simulink model "ACAES"  (R2026a)
settings: Solver=ode45  StopTime=t_sim_end  MaxStep=dt  MinStep=1  AbsTol=1e-6
model workspace (MAT data in the model file):
  Constant_mdot_ctrl = 0
  P0 = 101325
  P_comp_rated_W = 100000
  P_turb_rated_W = 100000
  T0 = 293.15
  buy_price = 15
  m_dot_chg_nom = 0.5
  m_dot_dis_nom = 0.6
  sell_price = 10
values from neighbouring files (symbols this model uses):
  cp_air = 1005.0    (= 1005)    [ACAES_params.m]    (also in ACAES_params.mat; CAES_init.m; IDKWHATTHISIS.mat)
  cp_TES = 2000    [ACAES_params.m]    (also in ACAES_params.mat; CAES_init.m = 1900; IDKWHATTHISIS.mat = 1900)
  cv_air = 717.95    [ACAES_params.m]    (also in ACAES_params.mat; CAES_init.m; IDKWHATTHISIS.mat)
  dP_HEX_frac = 0.005    [ACAES_params.m]    (also in ACAES_params.mat; CAES_init.m; IDKWHATTHISIS.mat)
  dt = t_vec(2) - t_vec(1)    [CAES_init.m]    (also in IDKWHATTHISIS.mat = 900)
  epsilon_HEX = 0.92    [ACAES_params.m]    (also in ACAES_params.mat; CAES_init.m = 0.9; IDKWHATTHISIS.mat = 0.9)
  eta_comp_vec = [0.55, 0.68, 0.78, 0.82, 0.82, 0.80, 0.74, 0.66, 0.55]    [CAES_init.m]    (also in IDKWHATTHISIS.mat = [0.55 0.68 0.78 0.82 0.82 0.8 0.74 0.66 0.55])
  eta_gen = 0.97    [ACAES_params.m]    (also in ACAES_params.mat; CAES_extract_results_annual.m = 0.96; CAES_init.m = 0.96; IDKWHATTHISIS.mat = 0.96)
  eta_mech_comp = 0.97    [ACAES_params.m]    (also in ACAES_params.mat; CAES_init.m; IDKWHATTHISIS.mat)
  eta_mech_turb = 0.98    [ACAES_params.m]    (also in ACAES_params.mat; CAES_init.m; IDKWHATTHISIS.mat)
  eta_motor = 0.96    [ACAES_params.m]    (also in ACAES_params.mat; CAES_init.m = 0.95; IDKWHATTHISIS.mat = 0.95)
  eta_turb_vec = [0.65, 0.75, 0.82, 0.85, 0.85, 0.83, 0.79, 0.73, 0.65]    [CAES_init.m]    (also in IDKWHATTHISIS.mat = [0.65 0.75 0.82 0.85 0.85 0.83 0.79 0.73 0.65])
  gamma = 1.4    [ACAES_params.m]    (also in ACAES_params.mat; CAES_init.m; IDKWHATTHISIS.mat)
  Kv_throttle = 0.01    [ACAES_params.m]    (also in ACAES_params.mat; CAES_init.m = 0.005; IDKWHATTHISIS.mat = 0.005)
  leakage_frac = 0.005    [ACAES_params.m]    (also in ACAES_params.mat; CAES_init.m = 0.003; IDKWHATTHISIS.mat = 0.003)
  m_hp_init = P_hp_min*V_hp/(R_air*T0)    (= 47534.8952924)    [ACAES_params.m]    (also in ACAES_params.mat; CAES_init.m = 23767.4476462; IDKWHATTHISIS.mat = 23767.4476462)
  m_TES = 5000    [ACAES_params.m]    (also in ACAES_params.mat; CAES_init.m = 2000; IDKWHATTHISIS.mat = 2000)
  N_stages = 3    [ACAES_params.m]    (also in ACAES_params.mat; CAES_init.m; IDKWHATTHISIS.mat)
  P_hp_init = P_hp_min    (= 4000000)    [ACAES_params.m]    (also in ACAES_params.mat; CAES_init.m; IDKWHATTHISIS.mat)
  P_hp_max = 7e6    (= 7000000)    [ACAES_params.m]    (also in ACAES_params.mat; CAES_init.m; IDKWHATTHISIS.mat)
  P_hp_min = 4e6    (= 4000000)    [ACAES_params.m]    (also in ACAES_params.mat; CAES_init.m; IDKWHATTHISIS.mat)
  P_net_discharge_thresh = 50000    [CAES_init.m]    (also in IDKWHATTHISIS.mat = 5000)
  P_throttle = 4e6    (= 4000000)    [ACAES_params.m]    (also in ACAES_params.mat; CAES_init.m; IDKWHATTHISIS.mat)
  PR_vec = [1.0 1.5 2.0 2.5 3.0 3.5 4.0 4.5 5.0]    [ACAES_params.m]    (also in ACAES_params.mat = [1 1.5 2 2.5 3 3.5 4 4.5 5]; CAES_init.m = [1.0, 1.5, 2.0, 2.5, 3.0, 3.5, 4.0, 4.5, 5.0]; IDKWHATTHISIS.mat = [1 1.5 2 2.5 3 3.5 4 4.5 5])
  R_air = 287.05    [ACAES_params.m]    (also in ACAES_params.mat; CAES_init.m; IDKWHATTHISIS.mat)
  SOC_hp_charge_start = 0.05    [CAES_init.m]    (also in IDKWHATTHISIS.mat)
  SOC_hp_charge_stop = 0.95    [CAES_init.m]    (also in IDKWHATTHISIS.mat)
  SOC_TES_discharge_min = 0.10    (= 0.1)    [CAES_init.m]    (also in IDKWHATTHISIS.mat)
  T_hp_init = T0    (= 293.15)    [ACAES_params.m]    (also in ACAES_params.mat; CAES_init.m; IDKWHATTHISIS.mat)
  T_TES_max = 500    [ACAES_params.m]    (also in ACAES_params.mat; CAES_init.m = 573.15; IDKWHATTHISIS.mat = 573.15)
  tau_valve = 0.5    [ACAES_params.m]    (also in ACAES_params.mat; CAES_init.m = 30; IDKWHATTHISIS.mat = 30)
  UA_TES_wall = 1.5    [CAES_init.m]    (also in IDKWHATTHISIS.mat)
  V_hp = 1000    [ACAES_params.m]    (also in ACAES_params.mat; CAES_init.m = 500; IDKWHATTHISIS.mat = 500)
undefined symbols (not defined in the file or in its folder): DiscIntNeverNeededParam
(part 1 of 2)
settings Model: Creator=amilcza  LastModifiedBy=amilcza

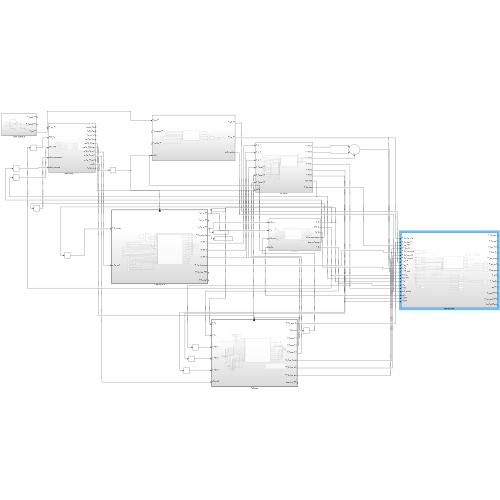
[thumbnail: Simulink's stored preview of the top-level diagram]
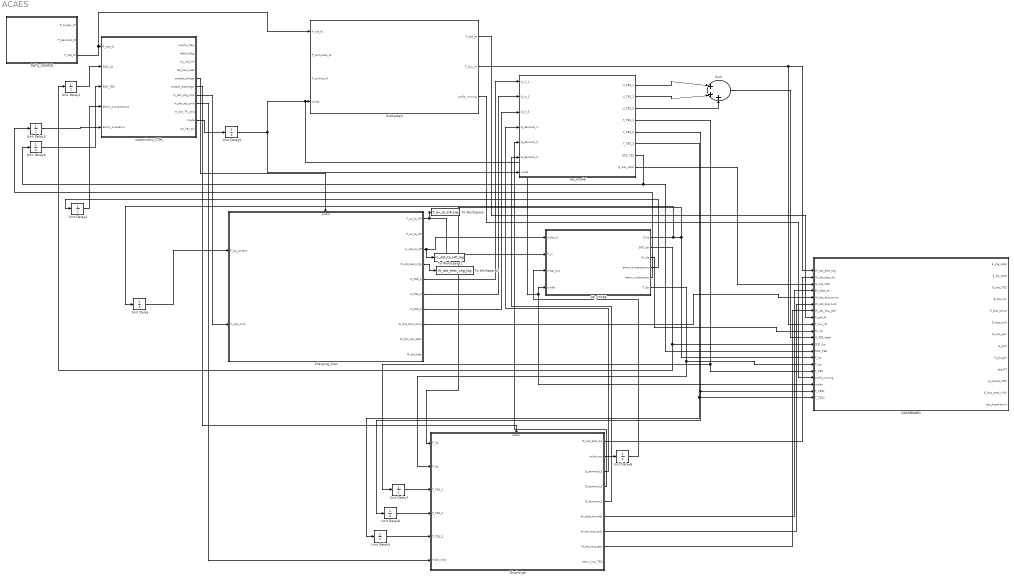
== system ACAES ==
  Charging_train : Subsystem
  DASHBOARD : Subsystem
  DATA_SOURCE : Subsystem
  Discharge : Subsystem
  HP_STORE : Subsystem
  Subsystem : Subsystem
  Sum : Sum  Inputs=|+++
  To Workspace : ToWorkspace  VariableName=T_air_to_HP_log  SaveFormat=Timeseries  SampleTime=-1
  To Workspace1 : ToWorkspace  VariableName=m_dot_to_HP_log  SaveFormat=Timeseries  SampleTime=-1
  To Workspace2 : ToWorkspace  VariableName=W_dot_elec_chg_log  SaveFormat=Timeseries  SampleTime=-1
  Unit Delay : UnitDelay  InitialCondition=P_hp_min  SampleTime=dt
  Unit Delay{1..6} (6 alike) : UnitDelay  SampleTime=dt
  Unit Delay7 : UnitDelay  InitialCondition=T0  SampleTime=dt
  Unit Delay8 : UnitDelay  InitialCondition=T0  SampleTime=dt
  Unit Delay9 : UnitDelay  InitialCondition=T0  SampleTime=dt
  supervisory_CTRL : Subsystem
  tes_model : Subsystem
  wires:
  DATA_SOURCE/3(P_net_W) -> Subsystem/1(P_net_W), supervisory_CTRL/1(P_net_W)
  supervisory_CTRL/10(mode) -> Unit Delay5/1
  supervisory_CTRL/8(m_dot_dis_cmd) -> Discharge/6(mdot_cmd)
  HP_STORE/4(alarm_overpressure) -> Unit Delay2/1
  Charging_train/1(T_air_to_HP) -> To Workspace/1, HP_STORE/2(T_in)
  Charging_train/3(m_dot_to_HP) -> To Workspace1/1, HP_STORE/1(mdot_in)
  Subsystem/3(profit_running) -> DASHBOARD/17(profit_running)
  Subsystem/2(P_buy_W) -> DASHBOARD/9(P_buy_W), DASHBOARD/1(W_dot_elec_chg)
  tes_model/5(T_TES_2) -> Unit Delay8/1, DASHBOARD/19(T_TES1)
  tes_model/6(T_TES_3) -> Unit Delay9/1, DASHBOARD/20(T_TES2)
  Subsystem/1(P_sell_W) -> DASHBOARD/8("P_sell_W  ")
  supervisory_CTRL/5(enable_charge) -> Charging_train/Enable
  supervisory_CTRL/6(enable_discharge) -> Discharge/Enable
  supervisory_CTRL/7(m_dot_chg_cmd) -> Charging_train/2(m_dot_cmd)
  HP_STORE/1(P_hp) -> Unit Delay/1, DASHBOARD/14(P_hp), Discharge/1(P_hp)
  HP_STORE/6(T_hp) -> Discharge/2(T_hp), DASHBOARD/15(T_hp)
  HP_STORE/2(SOC_hp) -> Unit Delay1/1, DASHBOARD/12(SOC_hp)
  tes_model/4(T_TES_1) -> DASHBOARD/16(T_TES), Unit Delay7/1
  tes_model/7(SOC_TES) -> Unit Delay4/1, DASHBOARD/13(SOC_TES)
  tes_model/8(Q_loss_total) -> DASHBOARD/3(Q_loss_TES)
  tes_model/1(U_TES_1) -> Sum/1
  tes_model/3(U_TES_3) -> Sum/3
  tes_model/2(U_TES_2) -> Sum/2
  Sum/1 -> DASHBOARD/11(U_TES_total)
  HP_STORE/3(Ex_hp) -> DASHBOARD/10(Ex_hp)
  Discharge/2(mdot_out) -> Unit Delay6/1
  Discharge/1(W_dot_elec_dis) -> DASHBOARD/2(W_dot_elec_dis)
  Discharge/3(Q_demand_1) -> tes_model/4(Q_demand_1)
  Discharge/4(Q_demand_2) -> tes_model/5(Q_demand_2)
  Discharge/5(Q_demand_3) -> tes_model/6(Q_demand_3)
  Discharge/6(Ex_dest_throttle) -> DASHBOARD/4(EX_dest_thr)
  Discharge/7(W_dot_loss_turb) -> DASHBOARD/6(W_dot_loss_turb)
  Discharge/8(W_dot_loss_gen) -> DASHBOARD/7(W_dot_loss_gen)
  Charging_train/8(W_dot_loss_comp) -> DASHBOARD/5(W_dot_loss_comp)
  Charging_train/5(Q_TES_1) -> tes_model/1(Q_in_1)
  Charging_train/6(Q_TES_2) -> tes_model/2(Q_in_2)
  Charging_train/7(Q_TES_3) -> tes_model/3(Q_in_3)
  Unit Delay/1 -> Charging_train/1(P_hp_current)
  Unit Delay1/1 -> supervisory_CTRL/2(SOC_hp)
  Unit Delay2/1 -> supervisory_CTRL/4(alarm_overpressure)
  Unit Delay4/1 -> supervisory_CTRL/3(SOC_TES)
  HP_STORE/5(alarm_undertemp) -> Unit Delay3/1
  Unit Delay3/1 -> supervisory_CTRL/5(alarm_overtemp)
  Unit Delay5/1 -> DASHBOARD/18(mode), HP_STORE/4(mode), Subsystem/4(mode), tes_model/7(mode)
  Unit Delay6/1 -> HP_STORE/3(mdot_out)
  Unit Delay7/1 -> Discharge/3(T_TES_1)
  Unit Delay8/1 -> Discharge/4(T_TES_2)
  Unit Delay9/1 -> Discharge/5(T_TES_3)
  Charging_train/4(W_dot_elec_chg) -> To Workspace2/1

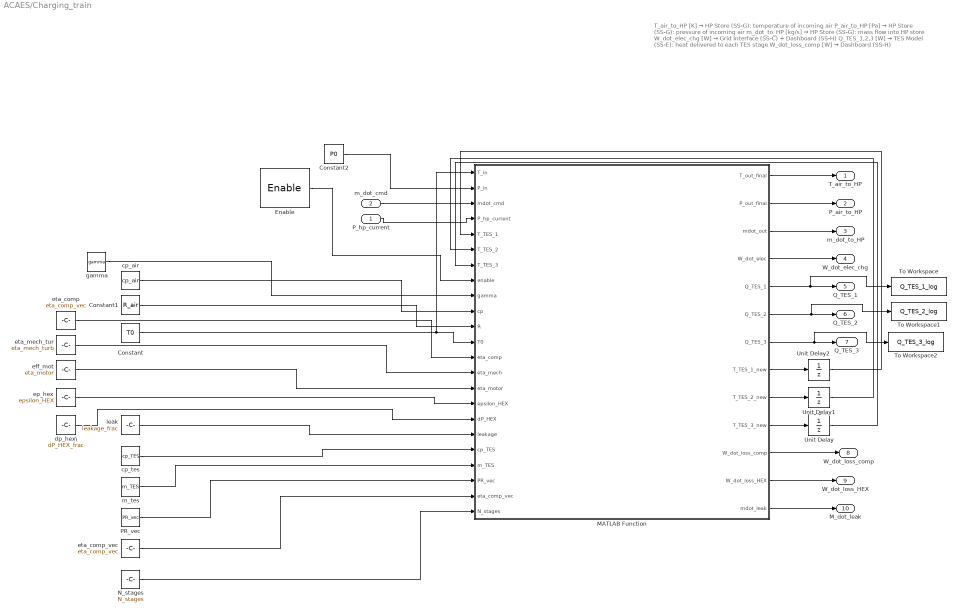
== system ACAES/Charging_train ==
  note: T_air_to_HP     [K]    → HP Store (SS-G): temperature of incoming air
      | P_air_to_HP     [Pa]   → HP Store (SS-G): pressure of incoming air
      | m_dot_to_HP     [kg/s] → HP Store (SS-G): mass flow into HP store
      | W_dot_elec_chg  [W]    → Grid Interface (SS-C) + Dashboard (SS-H)
      | Q_TES_1,2,3     [W]    → TES Model (SS-E): heat delivered to each TES stage
      | W_dot_loss_comp [W]    → Dashboard (SS-H)
  P_hp_current : Inport  SampleTime=dt
  m_dot_cmd : Inport  Port=2  SampleTime=dt
  Enable : EnablePort  PropagateVarSize=During execution  ShowOutputPort=on
  Constant : Constant  Value=T0  SampleTime=dt
  Constant1 : Constant  Value=R_air  SampleTime=dt
  Constant2 : Constant  Value=P0  SampleTime=dt
  MATLAB Function : MATLAB Function  TreatAsAtomicUnit=on
  N_stages : Constant  Value=N_stages  SampleTime=dt
  PR_vec : Constant  Value=PR_vec  SampleTime=dt
  To Workspace : ToWorkspace  VariableName=Q_TES_1_log  SaveFormat=Timeseries  SampleTime=-1
  To Workspace1 : ToWorkspace  VariableName=Q_TES_2_log  SaveFormat=Timeseries  SampleTime=-1
  To Workspace2 : ToWorkspace  VariableName=Q_TES_3_log  SaveFormat=Timeseries  SampleTime=-1
  Unit Delay : UnitDelay  InitialCondition=T0  SampleTime=dt
  Unit Delay1 : UnitDelay  InitialCondition=T0  SampleTime=dt
  Unit Delay2 : UnitDelay  InitialCondition=T0  SampleTime=dt
  cp_air : Constant  Value=cp_air  SampleTime=dt
  cp_tes : Constant  Value=cp_TES  SampleTime=dt
  dp_hex\ : Constant  Value=dP_HEX_frac  SampleTime=dt
  eff_mot : Constant  Value=eta_motor  SampleTime=dt
  ep_hex : Constant  Value=epsilon_HEX  SampleTime=dt
  eta_comp : Constant  Value=eta_comp_vec  SampleTime=dt
  eta_comp_vec : Constant  Value=eta_comp_vec  SampleTime=dt
  eta_mech_tur : Constant  Value=eta_mech_turb  SampleTime=dt
  gamma : Constant  Value=gamma  SampleTime=dt
  leak : Constant  Value=leakage_frac  SampleTime=dt
  m_tes : Constant  Value=m_TES  SampleTime=dt
  T_air_to_HP : Outport
  P_air_to_HP : Outport  Port=2
  m_dot_to_HP : Outport  Port=3
  W_dot_elec_chg : Outport  Port=4
  Q_TES_1 : Outport  Port=5
  Q_TES_2 : Outport  Port=6
  Q_TES_3 : Outport  Port=7
  W_dot_loss_comp : Outport  Port=8
  W_dot_loss_HEX : Outport  Port=9
  M_dot_leak : Outport  Port=10
  wires:
  N_stages/1 -> MATLAB Function/23(N_stages)
  eta_comp_vec/1 -> MATLAB Function/22(eta_comp_vec)
  PR_vec/1 -> MATLAB Function/21(PR_vec)
  m_tes/1 -> MATLAB Function/20(m_TES)
  cp_tes/1 -> MATLAB Function/19(cp_TES)
  leak/1 -> MATLAB Function/18(leakage)
  dp_hex\/1 -> MATLAB Function/17(dP_HEX)
  ep_hex/1 -> MATLAB Function/16(epsilon_HEX)
  eff_mot/1 -> MATLAB Function/15(eta_motor)
  eta_mech_tur/1 -> MATLAB Function/14(eta_mech)
  eta_comp/1 -> MATLAB Function/13(eta_comp)
  Constant/1 -> MATLAB Function/12(T0), MATLAB Function/1(T_in)
  Constant1/1 -> MATLAB Function/11(R)
  cp_air/1 -> MATLAB Function/10(cp)
  gamma/1 -> MATLAB Function/9(gamma)
  P_hp_current/1 -> MATLAB Function/4(P_hp_current)
  m_dot_cmd/1 -> MATLAB Function/3(mdot_cmd)
  MATLAB Function/1(T_out_final) -> T_air_to_HP/1
  MATLAB Function/2(P_out_final) -> P_air_to_HP/1
  MATLAB Function/3(mdot_out) -> m_dot_to_HP/1
  MATLAB Function/4(W_dot_elec) -> W_dot_elec_chg/1
  MATLAB Function/5(Q_TES_1) -> To Workspace/1, Q_TES_1/1
  MATLAB Function/6(Q_TES_2) -> To Workspace1/1, Q_TES_2/1
  MATLAB Function/7(Q_TES_3) -> To Workspace2/1, Q_TES_3/1
  MATLAB Function/11(W_dot_loss_comp) -> W_dot_loss_comp/1
  Enable/1 -> MATLAB Function/8(enable)
  MATLAB Function/12(W_dot_loss_HEX) -> W_dot_loss_HEX/1
  MATLAB Function/13(mdot_leak) -> M_dot_leak/1
  Constant2/1 -> MATLAB Function/2(P_in)
  MATLAB Function/10(T_TES_3_new) -> Unit Delay/1
  MATLAB Function/9(T_TES_2_new) -> Unit Delay1/1
  MATLAB Function/8(T_TES_1_new) -> Unit Delay2/1
  Unit Delay2/1 -> MATLAB Function/5(T_TES_1)
  Unit Delay1/1 -> MATLAB Function/6(T_TES_2)
  Unit Delay/1 -> MATLAB Function/7(T_TES_3)

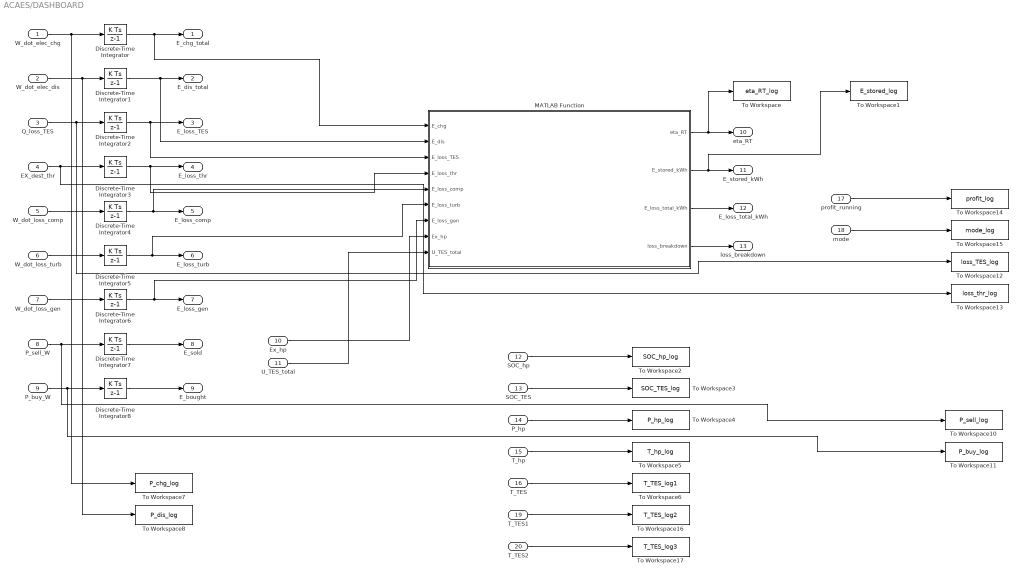
== system ACAES/DASHBOARD ==
  W_dot_elec_chg : Inport  SampleTime=dt
  W_dot_elec_dis : Inport  Port=2  SampleTime=dt
  Q_loss_TES : Inport  Port=3  SampleTime=dt
  EX_dest_thr : Inport  Port=4  SampleTime=dt
  W_dot_loss_comp : Inport  Port=5  SampleTime=dt
  W_dot_loss_turb : Inport  Port=6  SampleTime=dt
  W_dot_loss_gen : Inport  Port=7  SampleTime=dt
  "P_sell_W  " : Inport  Port=8  SampleTime=dt
  P_buy_W : Inport  Port=9  SampleTime=dt
  Ex_hp : Inport  Port=10  SampleTime=dt
  U_TES_total : Inport  Port=11  SampleTime=dt
  SOC_hp : Inport  Port=12  SampleTime=dt
  SOC_TES : Inport  Port=13  SampleTime=dt
  P_hp : Inport  Port=14  SampleTime=dt
  T_hp : Inport  Port=15  SampleTime=dt
  T_TES : Inport  Port=16  SampleTime=dt
  profit_running : Inport  Port=17  SampleTime=dt
  mode : Inport  Port=18  SampleTime=dt
  T_TES1 : Inport  Port=19  SampleTime=dt
  T_TES2 : Inport  Port=20  SampleTime=dt
  Discrete-Time Integrator{,1..8} (9 alike) : DiscreteIntegrator  SampleTime=dt  ICPrevOutput=DiscIntNeverNeededParam  ICPrevScaledInput=DiscIntNeverNeededParam
  MATLAB Function : MATLAB Function  TreatAsAtomicUnit=on
  To Workspace : ToWorkspace  VariableName=eta_RT_log  SaveFormat=Timeseries  SampleTime=-1
  To Workspace1 : ToWorkspace  VariableName=E_stored_log  SaveFormat=Timeseries  SampleTime=-1
  To Workspace10 : ToWorkspace  VariableName=P_sell_log  SaveFormat=Timeseries  SampleTime=-1
  To Workspace11 : ToWorkspace  VariableName=P_buy_log  SaveFormat=Timeseries  SampleTime=-1
  To Workspace12 : ToWorkspace  VariableName=loss_TES_log  SaveFormat=Timeseries  SampleTime=-1
  To Workspace13 : ToWorkspace  VariableName=loss_thr_log  SaveFormat=Timeseries  SampleTime=-1
  To Workspace14 : ToWorkspace  VariableName=profit_log  SaveFormat=Timeseries  SampleTime=-1
  To Workspace15 : ToWorkspace  VariableName=mode_log  SaveFormat=Timeseries  SampleTime=-1
  To Workspace16 : ToWorkspace  VariableName=T_TES_log2  SaveFormat=Timeseries  SampleTime=-1
  To Workspace17 : ToWorkspace  VariableName=T_TES_log3  SaveFormat=Timeseries  SampleTime=-1
  To Workspace2 : ToWorkspace  VariableName=SOC_hp_log  SaveFormat=Timeseries  SampleTime=-1
  To Workspace3 : ToWorkspace  VariableName=SOC_TES_log  SaveFormat=Timeseries  SampleTime=-1
  To Workspace4 : ToWorkspace  VariableName=P_hp_log  SaveFormat=Timeseries  SampleTime=-1
  To Workspace5 : ToWorkspace  VariableName=T_hp_log  SaveFormat=Timeseries  SampleTime=-1
  To Workspace6 : ToWorkspace  VariableName=T_TES_log1  SaveFormat=Timeseries  SampleTime=-1
  To Workspace7 : ToWorkspace  VariableName=P_chg_log  SaveFormat=Timeseries  SampleTime=-1
  To Workspace8 : ToWorkspace  VariableName=P_dis_log  SaveFormat=Timeseries  SampleTime=-1
  "E_chg_total " : Outport  Unit=J
  "E_dis_total " : Outport  Port=2  Unit=J
  E_loss_TES : Outport  Port=3  Unit=J
  E_loss_thr : Outport  Port=4  Unit=J
  E_loss_comp : Outport  Port=5  Unit=J
  E_loss_turb : Outport  Port=6
  E_loss_gen : Outport  Port=7  Unit=J
  E_sold : Outport  Port=8  Unit=J
  E_bought : Outport  Port=9  Unit=J
  eta_RT : Outport  Port=10
  E_stored_kWh : Outport  Port=11
  E_loss_total_kWh : Outport  Port=12
  loss_breakdown : Outport  Port=13
  wires:
  W_dot_elec_chg/1 -> To Workspace7/1, Discrete-Time Integrator/1
  W_dot_elec_dis/1 -> To Workspace8/1, Discrete-Time Integrator1/1
  Discrete-Time Integrator/1 -> MATLAB Function/1(E_chg), "E_chg_total "/1
  Discrete-Time Integrator1/1 -> MATLAB Function/2(E_dis), "E_dis_total "/1
  Discrete-Time Integrator2/1 -> MATLAB Function/3(E_loss_TES), E_loss_TES/1
  Q_loss_TES/1 -> To Workspace12/1, Discrete-Time Integrator2/1
  EX_dest_thr/1 -> To Workspace13/1, Discrete-Time Integrator3/1
  W_dot_loss_comp/1 -> Discrete-Time Integrator4/1
  W_dot_loss_turb/1 -> Discrete-Time Integrator5/1
  W_dot_loss_gen/1 -> Discrete-Time Integrator6/1
  "P_sell_W  "/1 -> To Workspace10/1, Discrete-Time Integrator7/1
  P_buy_W/1 -> To Workspace11/1, Discrete-Time Integrator8/1
  Discrete-Time Integrator3/1 -> MATLAB Function/4(E_loss_thr), E_loss_thr/1
  Discrete-Time Integrator4/1 -> MATLAB Function/5(E_loss_comp), E_loss_comp/1
  Discrete-Time Integrator5/1 -> MATLAB Function/6(E_loss_turb), E_loss_turb/1
  Discrete-Time Integrator6/1 -> MATLAB Function/7(E_loss_gen), E_loss_gen/1
  Discrete-Time Integrator7/1 -> E_sold/1
  Discrete-Time Integrator8/1 -> E_bought/1
  Ex_hp/1 -> MATLAB Function/8(Ex_hp)
  U_TES_total/1 -> MATLAB Function/9(U_TES_total)
  MATLAB Function/1(eta_RT) -> To Workspace/1, eta_RT/1
  MATLAB Function/2(E_stored_kWh) -> To Workspace1/1, E_stored_kWh/1
  MATLAB Function/3(E_loss_total_kWh) -> E_loss_total_kWh/1
  MATLAB Function/4(loss_breakdown) -> loss_breakdown/1
  SOC_hp/1 -> To Workspace2/1
  SOC_TES/1 -> To Workspace3/1
  P_hp/1 -> To Workspace4/1
  T_TES/1 -> To Workspace6/1
  T_hp/1 -> To Workspace5/1
  profit_running/1 -> To Workspace14/1
  mode/1 -> To Workspace15/1
  T_TES1/1 -> To Workspace16/1
  T_TES2/1 -> To Workspace17/1

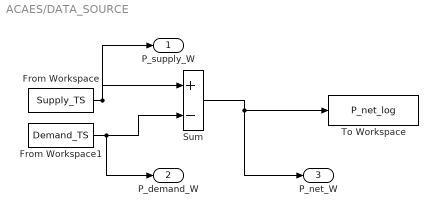
== system ACAES/DATA_SOURCE ==
  From Workspace : FromWorkspace  VariableName=Supply_TS  SampleTime=dt
  From Workspace1 : FromWorkspace  VariableName=Demand_TS  SampleTime=dt
  Sum : Sum  Inputs=|+-
  To Workspace : ToWorkspace  VariableName=P_net_log  SaveFormat=Timeseries  SampleTime=-1
  P_supply_W : Outport
  P_demand_W : Outport  Port=2
  P_net_W : Outport  Port=3
  wires:
  From Workspace/1 -> P_supply_W/1, Sum/1
  From Workspace1/1 -> P_demand_W/1, Sum/2
  Sum/1 -> P_net_W/1, To Workspace/1

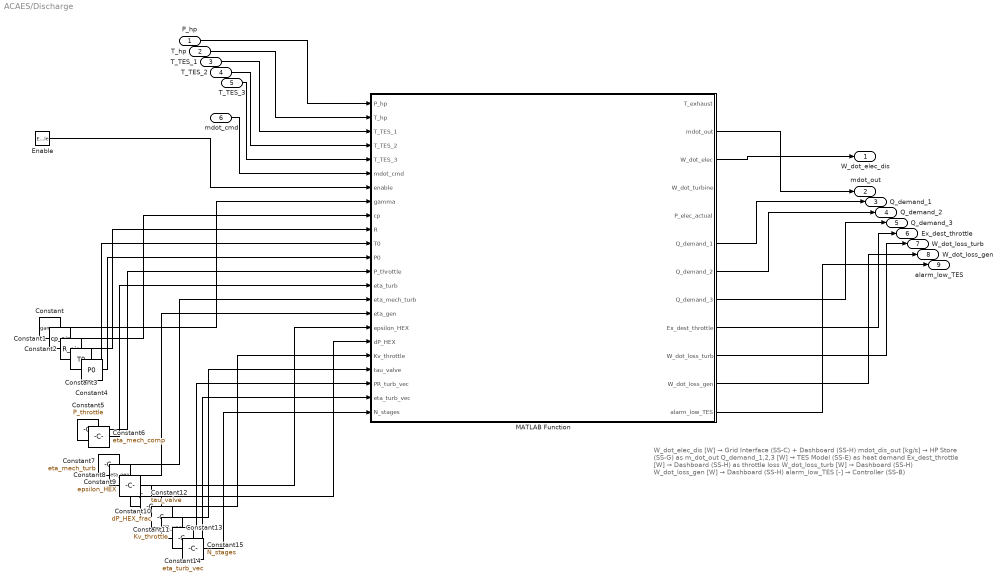
== system ACAES/Discharge ==
  note: W_dot_elec_dis   [W]    → Grid Interface (SS-C) + Dashboard (SS-H)
      | mdot_dis_out     [kg/s] → HP Store (SS-G) as m_dot_out
      | Q_demand_1,2,3   [W]    → TES Model (SS-E) as heat demand
      | Ex_dest_throttle [W]    → Dashboard (SS-H) as throttle loss
      | W_dot_loss_turb  [W]    → Dashboard (SS-H)
      | W_dot_loss_gen   [W]    → Dashboard (SS-H)
      | alarm_low_TES    [-]    → Controller (SS-B)
  P_hp : Inport  SampleTime=dt
  T_hp : Inport  Port=2  SampleTime=dt
  T_TES_1 : Inport  Port=3  SampleTime=dt
  T_TES_2 : Inport  Port=4  SampleTime=dt
  T_TES_3 : Inport  Port=5  SampleTime=dt
  mdot_cmd : Inport  Port=6  SampleTime=dt
  Enable : EnablePort  ShowOutputPort=on
  Constant : Constant  Value=gamma  SampleTime=dt
  Constant1 : Constant  Value=cp_air  SampleTime=dt
  Constant10 : Constant  Value=dP_HEX_frac  SampleTime=dt
  Constant11 : Constant  Value=Kv_throttle  SampleTime=dt
  Constant12 : Constant  Value=tau_valve  SampleTime=dt
  Constant13 : Constant  Value=PR_vec  SampleTime=dt
  Constant14 : Constant  Value=eta_turb_vec  SampleTime=dt
  Constant15 : Constant  Value=N_stages  SampleTime=dt
  Constant2 : Constant  Value=R_air  SampleTime=dt
  Constant3 : Constant  Value=T0  SampleTime=dt
  Constant4 : Constant  Value=P0  SampleTime=dt
  Constant5 : Constant  Value=P_throttle  SampleTime=dt
  Constant6 : Constant  Value=eta_mech_comp  SampleTime=dt
  Constant7 : Constant  Value=eta_mech_turb  SampleTime=dt
  Constant8 : Constant  Value=eta_gen  SampleTime=dt
  Constant9 : Constant  Value=epsilon_HEX  SampleTime=dt
  MATLAB Function : MATLAB Function  TreatAsAtomicUnit=on
  W_dot_elec_dis : Outport
  mdot_out : Outport  Port=2
  Q_demand_1 : Outport  Port=3
  Q_demand_2 : Outport  Port=4
  Q_demand_3 : Outport  Port=5
  Ex_dest_throttle : Outport  Port=6
  W_dot_loss_turb : Outport  Port=7
  W_dot_loss_gen : Outport  Port=8
  alarm_low_TES : Outport  Port=9
  wires:
  MATLAB Function/12(alarm_low_TES) -> alarm_low_TES/1
  MATLAB Function/11(W_dot_loss_gen) -> W_dot_loss_gen/1
  MATLAB Function/10(W_dot_loss_turb) -> W_dot_loss_turb/1
  MATLAB Function/9(Ex_dest_throttle) -> Ex_dest_throttle/1
  MATLAB Function/8(Q_demand_3) -> Q_demand_3/1
  MATLAB Function/7(Q_demand_2) -> Q_demand_2/1
  MATLAB Function/6(Q_demand_1) -> Q_demand_1/1
  MATLAB Function/2(mdot_out) -> mdot_out/1
  Enable/1 -> MATLAB Function/7(enable)
  Constant/1 -> MATLAB Function/8(gamma)
  Constant1/1 -> MATLAB Function/9(cp)
  Constant2/1 -> MATLAB Function/10(R)
  Constant3/1 -> MATLAB Function/11(T0)
  Constant4/1 -> MATLAB Function/12(P0)
  Constant5/1 -> MATLAB Function/13(P_throttle)
  Constant6/1 -> MATLAB Function/14(eta_turb)
  Constant7/1 -> MATLAB Function/15(eta_mech_turb)
  Constant8/1 -> MATLAB Function/16(eta_gen)
  Constant9/1 -> MATLAB Function/17(epsilon_HEX)
  Constant10/1 -> MATLAB Function/18(dP_HEX)
  Constant11/1 -> MATLAB Function/19(Kv_throttle)
  Constant12/1 -> MATLAB Function/20(tau_valve)
  Constant13/1 -> MATLAB Function/21(PR_turb_vec)
  Constant14/1 -> MATLAB Function/22(eta_turb_vec)
  Constant15/1 -> MATLAB Function/23(N_stages)
  P_hp/1 -> MATLAB Function/1(P_hp)
  T_hp/1 -> MATLAB Function/2(T_hp)
  T_TES_1/1 -> MATLAB Function/3(T_TES_1)
  T_TES_2/1 -> MATLAB Function/4(T_TES_2)
  T_TES_3/1 -> MATLAB Function/5(T_TES_3)
  mdot_cmd/1 -> MATLAB Function/6(mdot_cmd)
  MATLAB Function/3(W_dot_elec) -> W_dot_elec_dis/1

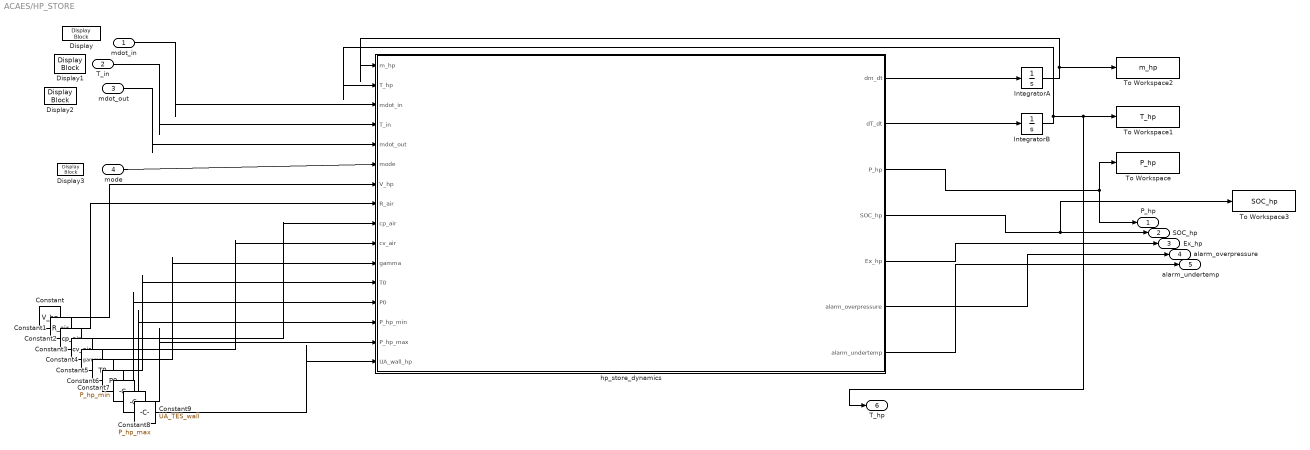
== system ACAES/HP_STORE ==
  mdot_in : Inport  SampleTime=dt
  T_in : Inport  Port=2  SampleTime=dt
  mdot_out : Inport  Port=3  SampleTime=dt
  mode : Inport  Port=4  SampleTime=dt
  Constant : Constant  Value=V_hp  SampleTime=dt
  Constant1 : Constant  Value=R_air  SampleTime=dt
  Constant2 : Constant  Value=cp_air  SampleTime=dt
  Constant3 : Constant  Value=cv_air  SampleTime=dt
  Constant4 : Constant  Value=gamma  SampleTime=dt
  Constant5 : Constant  Value=T0  SampleTime=dt
  Constant6 : Constant  Value=P0  SampleTime=dt
  Constant7 : Constant  Value=P_hp_min  SampleTime=dt
  Constant8 : Constant  Value=P_hp_max  SampleTime=dt
  Constant9 : Constant  Value=UA_TES_wall  SampleTime=dt
  Display{,1..3} (4 alike) : DisplayBlock  LabelPosition=Hide  Transparency=1  GridColor=[0.502, 0.502, 0.502]
  IntegratorA : Integrator  InitialCondition=m_hp_init
  IntegratorB : Integrator  InitialCondition=T_hp_init
  To Workspace : ToWorkspace  VariableName=P_hp  SaveFormat=Timeseries  SampleTime=-1
  To Workspace1 : ToWorkspace  VariableName=T_hp  SaveFormat=Timeseries  SampleTime=-1
  To Workspace2 : ToWorkspace  VariableName=m_hp  SaveFormat=Timeseries  SampleTime=-1
  To Workspace3 : ToWorkspace  VariableName=SOC_hp  SaveFormat=Timeseries  SampleTime=-1
  hp_store_dynamics : MATLAB Function  TreatAsAtomicUnit=on
  P_hp : Outport
  SOC_hp : Outport  Port=2
  Ex_hp : Outport  Port=3
  alarm_overpressure : Outport  Port=4
  alarm_undertemp : Outport  Port=5
  T_hp : Outport  Port=6
  wires:
  Constant/1 -> hp_store_dynamics/7(V_hp)
  Constant1/1 -> hp_store_dynamics/8(R_air)
  Constant2/1 -> hp_store_dynamics/9(cp_air)
  Constant3/1 -> hp_store_dynamics/10(cv_air)
  Constant4/1 -> hp_store_dynamics/11(gamma)
  Constant5/1 -> hp_store_dynamics/12(T0)
  Constant6/1 -> hp_store_dynamics/13(P0)
  Constant7/1 -> hp_store_dynamics/14(P_hp_min)
  Constant8/1 -> hp_store_dynamics/15(P_hp_max)
  Constant9/1 -> hp_store_dynamics/16(UA_wall_hp)
  T_in/1 -> hp_store_dynamics/4(T_in)
  mdot_out/1 -> hp_store_dynamics/5(mdot_out)
  mode/1 -> hp_store_dynamics/6(mode)
  hp_store_dynamics/1(dm_dt) -> IntegratorA/1
  hp_store_dynamics/2(dT_dt) -> IntegratorB/1
  hp_store_dynamics/6(alarm_overpressure) -> alarm_overpressure/1
  hp_store_dynamics/7(alarm_undertemp) -> alarm_undertemp/1
  hp_store_dynamics/5(Ex_hp) -> Ex_hp/1
  hp_store_dynamics/4(SOC_hp) -> To Workspace3/1, SOC_hp/1
  hp_store_dynamics/3(P_hp) -> P_hp/1, To Workspace/1
  IntegratorA/1 -> To Workspace2/1, hp_store_dynamics/1(m_hp)
  IntegratorB/1 -> T_hp/1, To Workspace1/1, hp_store_dynamics/2(T_hp)
  mdot_in/1 -> hp_store_dynamics/3(mdot_in)

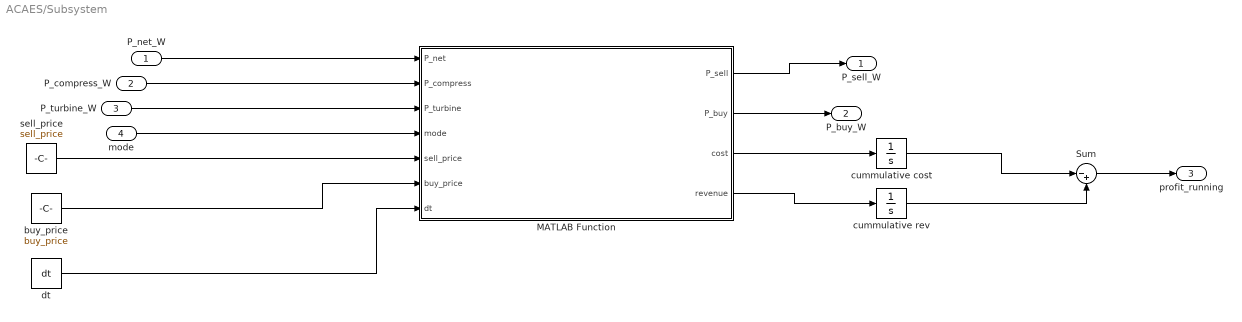
== system ACAES/Subsystem ==
  P_net_W : Inport  Unit=W  SampleTime=dt
  P_compress_W : Inport  Port=2  Unit=W  SampleTime=dt
  P_turbine_W : Inport  Port=3  Unit=W  SampleTime=dt
  mode : Inport  Port=4  SampleTime=dt
  MATLAB Function : MATLAB Function  TreatAsAtomicUnit=on
  Sum : Sum  Inputs=|-+
  buy_price : Constant  Value=buy_price  SampleTime=dt
  cummulative cost : Integrator
  cummulative rev : Integrator
  dt : Constant  Value=dt  SampleTime=dt
  sell_price : Constant  Value=sell_price  SampleTime=dt
  P_sell_W : Outport
  P_buy_W : Outport  Port=2
  profit_running : Outport  Port=3
  wires:
  P_compress_W/1 -> MATLAB Function/2(P_compress)
  P_turbine_W/1 -> MATLAB Function/3(P_turbine)
  P_net_W/1 -> MATLAB Function/1(P_net)
  mode/1 -> MATLAB Function/4(mode)
  sell_price/1 -> MATLAB Function/5(sell_price)
  buy_price/1 -> MATLAB Function/6(buy_price)
  dt/1 -> MATLAB Function/7(dt)
  MATLAB Function/4(revenue) -> cummulative rev/1
  MATLAB Function/3(cost) -> cummulative cost/1
  cummulative rev/1 -> Sum/2
  cummulative cost/1 -> Sum/1
  MATLAB Function/1(P_sell) -> P_sell_W/1
  MATLAB Function/2(P_buy) -> P_buy_W/1
  Sum/1 -> profit_running/1

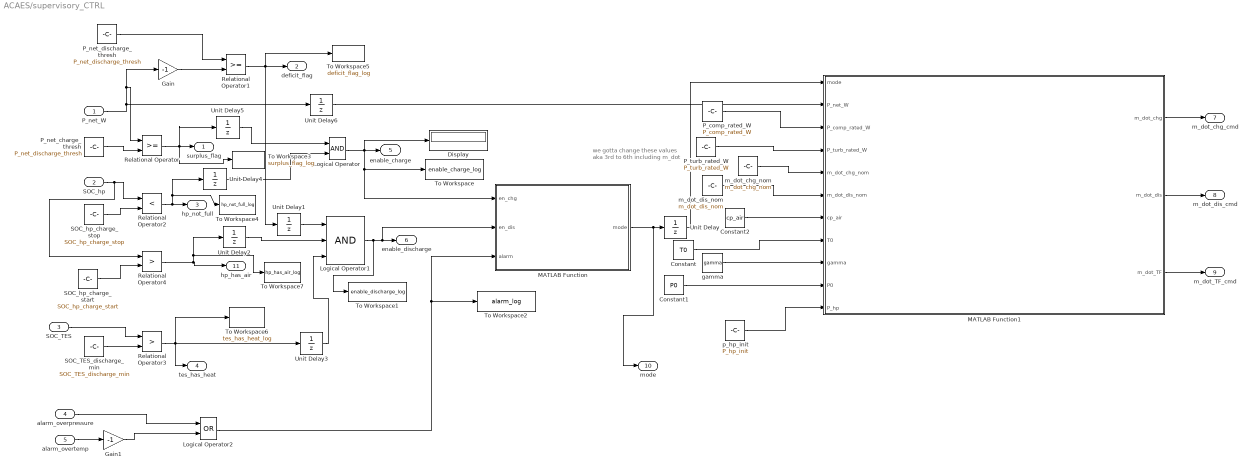
== system ACAES/supervisory_CTRL ==
  note: we gotta change these values
      | aka 3rd to 6th
      | including m_dot
  P_net_W : Inport  Unit=W  SampleTime=dt
  SOC_hp : Inport  Port=2  SampleTime=dt
  SOC_TES : Inport  Port=3  SampleTime=dt
  alarm_overpressure : Inport  Port=4  SampleTime=dt
  alarm_overtemp : Inport  Port=5  SampleTime=dt
  Constant : Constant  Value=T0  SampleTime=dt
  Constant1 : Constant  Value=P0  SampleTime=dt
  Constant2 : Constant  Value=cp_air  SampleTime=dt
  Display : Display
  Gain : Gain  Gain=-1
  Gain1 : Gain  Gain=-1
  Logical Operator : Logic  AllPortsSameDT=off  OutDataTypeStr=boolean
  Logical Operator1 : Logic  Inputs=3  AllPortsSameDT=off  OutDataTypeStr=boolean
  Logical Operator2 : Logic  Operator=OR  AllPortsSameDT=off  OutDataTypeStr=boolean
  MATLAB Function : MATLAB Function  TreatAsAtomicUnit=on
  MATLAB Function1 : MATLAB Function  TreatAsAtomicUnit=on
  P_comp_rated_W : Constant  Value=P_comp_rated_W  SampleTime=dt
  P_net_charge_thresh : Constant  Value=P_net_discharge_thresh  SampleTime=dt
  P_net_discharge_thresh : Constant  Value=P_net_discharge_thresh  SampleTime=dt
  P_turb_rated_W : Constant  Value=P_turb_rated_W  SampleTime=dt
  Relational Operator : RelationalOperator  OutDataTypeStr=boolean  RndMeth=Simplest  InputSameDT=off
  Relational Operator1 : RelationalOperator  OutDataTypeStr=boolean  RndMeth=Simplest  InputSameDT=off
  Relational Operator2 : RelationalOperator  Operator=<  OutDataTypeStr=boolean  RndMeth=Simplest  InputSameDT=off
  Relational Operator3 : RelationalOperator  Operator=>  OutDataTypeStr=boolean  RndMeth=Simplest  InputSameDT=off
  Relational Operator4 : RelationalOperator  Operator=>  OutDataTypeStr=boolean  RndMeth=Simplest  InputSameDT=off
  SOC_TES_discharge_min : Constant  Value=SOC_TES_discharge_min  SampleTime=dt
  SOC_hp_charge_start : Constant  Value=SOC_hp_charge_start  SampleTime=dt
  SOC_hp_charge_stop : Constant  Value=SOC_hp_charge_stop  SampleTime=dt
  To Workspace : ToWorkspace  VariableName=enable_charge_log  SaveFormat=Timeseries  SampleTime=-1
  To Workspace1 : ToWorkspace  VariableName=enable_discharge_log  SaveFormat=Timeseries  SampleTime=-1
  To Workspace2 : ToWorkspace  VariableName=alarm_log  SaveFormat=Timeseries  SampleTime=-1
  To Workspace3 : ToWorkspace  VariableName=surplus_flag_log  SaveFormat=Timeseries  SampleTime=-1
  To Workspace4 : ToWorkspace  VariableName=hp_not_full_log  SaveFormat=Timeseries  SampleTime=-1
  To Workspace5 : ToWorkspace  VariableName=deficit_flag_log  SaveFormat=Timeseries  SampleTime=-1
  To Workspace6 : ToWorkspace  VariableName=tes_has_heat_log  SaveFormat=Timeseries  SampleTime=-1
  To Workspace7 : ToWorkspace  VariableName=hp_has_air_log  SaveFormat=Timeseries  SampleTime=-1
  Unit Delay{,1..6} (7 alike) : UnitDelay  SampleTime=dt
  gamma : Constant  Value=gamma  SampleTime=dt
  m_dot_chg_nom : Constant  Value=m_dot_chg_nom  SampleTime=dt
  m_dot_dis_nom : Constant  Value=m_dot_dis_nom  SampleTime=dt
  p_hp_init : Constant  Value=P_hp_init  SampleTime=dt
  surplus_flag : Outport
  deficit_flag : Outport  Port=2
  hp_not_full : Outport  Port=3
  tes_has_heat : Outport  Port=4
  enable_charge : Outport  Port=5
  enable_discharge : Outport  Port=6
  m_dot_chg_cmd : Outport  Port=7
  m_dot_dis_cmd : Outport  Port=8
  m_dot_TF_cmd : Outport  Port=9
  mode : Outport  Port=10
  hp_has_air : Outport  Port=11
  wires:
  P_net_W/1 -> Unit Delay6/1, Gain/1, Relational Operator/1
  P_net_charge_thresh/1 -> Relational Operator/2
  Relational Operator/1 -> To Workspace3/1, Unit Delay5/1, surplus_flag/1
  Gain/1 -> Relational Operator1/2
  P_net_discharge_thresh/1 -> Relational Operator1/1
  Relational Operator1/1 -> To Workspace5/1, Unit Delay1/1, deficit_flag/1
  SOC_hp_charge_stop/1 -> Relational Operator2/2
  SOC_hp/1 -> Relational Operator4/1, Relational Operator2/1
  Relational Operator2/1 -> To Workspace4/1, Unit Delay4/1, hp_not_full/1
  SOC_TES_discharge_min/1 -> Relational Operator3/2
  SOC_TES/1 -> Relational Operator3/1
  Relational Operator3/1 -> To Workspace6/1, tes_has_heat/1, Unit Delay3/1
  Logical Operator/1 -> To Workspace/1, MATLAB Function/1(en_chg), Display/1, enable_charge/1
  Logical Operator1/1 -> MATLAB Function/2(en_dis), enable_discharge/1, To Workspace1/1
  Logical Operator2/1 -> To Workspace2/1, MATLAB Function/3(alarm)
  alarm_overpressure/1 -> Logical Operator2/1
  alarm_overtemp/1 -> Gain1/1
  MATLAB Function1/1(m_dot_chg) -> m_dot_chg_cmd/1
  MATLAB Function1/2(m_dot_dis) -> m_dot_dis_cmd/1
  MATLAB Function1/3(m_dot_TF) -> m_dot_TF_cmd/1
  MATLAB Function/1(mode) -> mode/1, Unit Delay/1
  Constant/1 -> MATLAB Function1/8(T0)
  Constant1/1 -> MATLAB Function1/10(P0)
  gamma/1 -> MATLAB Function1/9(gamma)
  Constant2/1 -> MATLAB Function1/7(cp_air)
  p_hp_init/1 -> MATLAB Function1/11(P_hp)
  m_dot_chg_nom/1 -> MATLAB Function1/5(m_dot_chg_nom)
  m_dot_dis_nom/1 -> MATLAB Function1/6(m_dot_dis_nom)
  P_comp_rated_W/1 -> MATLAB Function1/3(P_comp_rated_W)
  P_turb_rated_W/1 -> MATLAB Function1/4(P_turb_rated_W)
  Gain1/1 -> Logical Operator2/2
  Unit Delay/1 -> MATLAB Function1/1(mode)
  Unit Delay1/1 -> Logical Operator1/1
  Unit Delay3/1 -> Logical Operator1/3
  Unit Delay4/1 -> Logical Operator/2
  Unit Delay5/1 -> Logical Operator/1
  Unit Delay6/1 -> MATLAB Function1/2(P_net_W)
  SOC_hp_charge_start/1 -> Relational Operator4/2
  Relational Operator4/1 -> To Workspace7/1, Unit Delay2/1, hp_has_air/1
  Unit Delay2/1 -> Logical Operator1/2

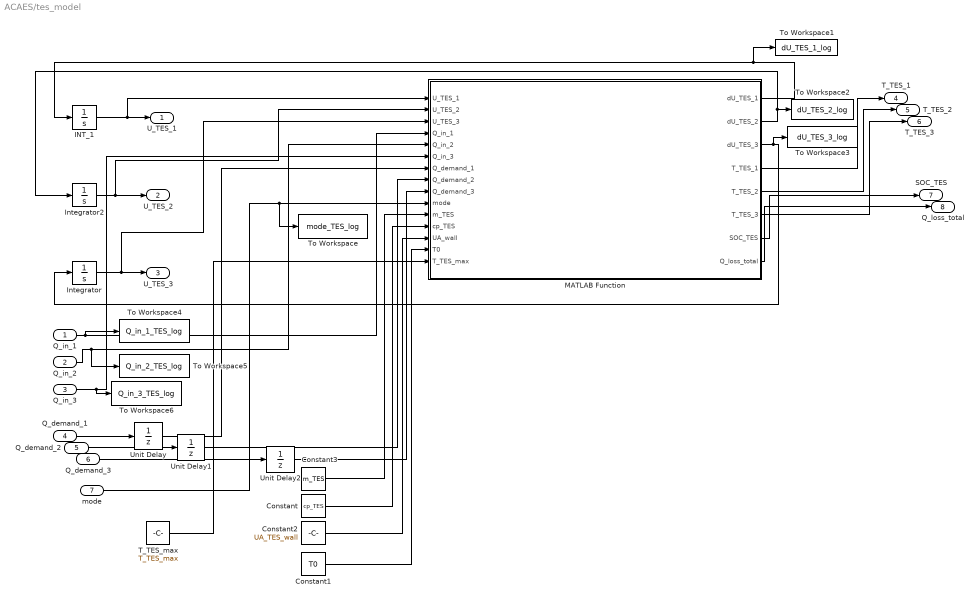
== system ACAES/tes_model ==
  Q_in_1 : Inport  SampleTime=dt
  Q_in_2 : Inport  Port=2  SampleTime=dt
  Q_in_3 : Inport  Port=3  SampleTime=dt
  Q_demand_1 : Inport  Port=4  SampleTime=dt
  Q_demand_2 : Inport  Port=5  SampleTime=dt
  Q_demand_3 : Inport  Port=6  SampleTime=dt
  mode : Inport  Port=7  SampleTime=dt
  Constant : Constant  Value=cp_TES  SampleTime=dt
  Constant1 : Constant  Value=T0  SampleTime=dt
  Constant2 : Constant  Value=UA_TES_wall  SampleTime=dt
  Constant3 : Constant  Value=m_TES  SampleTime=dt
  INT_1 : Integrator  InitialCondition=T0 * m_TES * cp_TES
  Integrator : Integrator  InitialCondition=T0 * m_TES * cp_TES
  Integrator2 : Integrator  InitialCondition=T0 * m_TES * cp_TES
  MATLAB Function : MATLAB Function  TreatAsAtomicUnit=on
  T_TES_max : Constant  Value=T_TES_max  SampleTime=dt
  To Workspace : ToWorkspace  VariableName=mode_TES_log  SaveFormat=Timeseries  SampleTime=-1
  To Workspace1 : ToWorkspace  VariableName=dU_TES_1_log  SaveFormat=Timeseries  SampleTime=-1
  To Workspace2 : ToWorkspace  VariableName=dU_TES_2_log  SaveFormat=Timeseries  SampleTime=-1
  To Workspace3 : ToWorkspace  VariableName=dU_TES_3_log  SaveFormat=Timeseries  SampleTime=-1
  To Workspace4 : ToWorkspace  VariableName=Q_in_1_TES_log  SaveFormat=Timeseries  SampleTime=-1
  To Workspace5 : ToWorkspace  VariableName=Q_in_2_TES_log  SaveFormat=Timeseries  SampleTime=-1
  To Workspace6 : ToWorkspace  VariableName=Q_in_3_TES_log  SaveFormat=Timeseries  SampleTime=-1
  Unit Delay : UnitDelay  SampleTime=dt
  Unit Delay1 : UnitDelay  SampleTime=dt
  Unit Delay2 : UnitDelay  SampleTime=dt
  U_TES_1 : Outport
  U_TES_2 : Outport  Port=2
  U_TES_3 : Outport  Port=3
  T_TES_1 : Outport  Port=4
  T_TES_2 : Outport  Port=5
  T_TES_3 : Outport  Port=6
  SOC_TES : Outport  Port=7
  Q_loss_total : Outport  Port=8
  wires:
  INT_1/1 -> MATLAB Function/1(U_TES_1), U_TES_1/1
  Integrator2/1 -> MATLAB Function/2(U_TES_2), U_TES_2/1
  Integrator/1 -> MATLAB Function/3(U_TES_3), U_TES_3/1
  MATLAB Function/1(dU_TES_1) -> To Workspace1/1, INT_1/1
  MATLAB Function/2(dU_TES_2) -> Integrator2/1, To Workspace2/1
  MATLAB Function/3(dU_TES_3) -> To Workspace3/1, Integrator/1
  Constant/1 -> MATLAB Function/12(cp_TES)
  Constant1/1 -> MATLAB Function/14(T0)
  Constant2/1 -> MATLAB Function/13(UA_wall)
  Constant3/1 -> MATLAB Function/11(m_TES)
  Q_in_1/1 -> To Workspace4/1, MATLAB Function/4(Q_in_1)
  Q_in_2/1 -> To Workspace5/1, MATLAB Function/5(Q_in_2)
  Q_in_3/1 -> To Workspace6/1, MATLAB Function/6(Q_in_3)
  Q_demand_1/1 -> Unit Delay/1
  Q_demand_2/1 -> Unit Delay1/1
  Q_demand_3/1 -> Unit Delay2/1
  mode/1 -> MATLAB Function/10(mode), To Workspace/1
  T_TES_max/1 -> MATLAB Function/15(T_TES_max)
  MATLAB Function/4(T_TES_1) -> T_TES_1/1
  MATLAB Function/5(T_TES_2) -> T_TES_2/1
  MATLAB Function/6(T_TES_3) -> T_TES_3/1
  MATLAB Function/7(SOC_TES) -> SOC_TES/1
  MATLAB Function/8(Q_loss_total) -> Q_loss_total/1
  Unit Delay/1 -> MATLAB Function/7(Q_demand_1)
  Unit Delay1/1 -> MATLAB Function/8(Q_demand_2)
  Unit Delay2/1 -> MATLAB Function/9(Q_demand_3)

== matlab function ACAES/tes_model/MATLAB Function ==
  data: U_TES_1 input; dU_TES_1 output; U_TES_2 input; U_TES_3 input; Q_in_1 input; Q_in_2 input; Q_in_3 input; Q_demand_1 input; Q_demand_2 input; Q_demand_3 input; mode input; m_TES input; cp_TES input; UA_wall input; T0 input; T_TES_max input; dU_TES_2 output; dU_TES_3 output; T_TES_1 output; T_TES_2 output; T_TES_3 output; SOC_TES output; Q_loss_total output
function [dU_TES_1, dU_TES_2, dU_TES_3, T_TES_1, T_TES_2, T_TES_3, ...
          SOC_TES, Q_loss_total] = ...
    TES_dynamics(U_TES_1, U_TES_2, U_TES_3, ...
                 Q_in_1, Q_in_2, Q_in_3, ...
                 Q_demand_1, Q_demand_2, Q_demand_3, ...
                 mode, m_TES, cp_TES, UA_wall, T0, T_TES_max)
% TES_DYNAMICS: First-law energy balance for 3-stage thermal store
%
% CHARGING (mode=1): Q_in from HEX goes into each TES stage
%                    dU_i = Q_in_i - Q_loss_i
%
% IDLE (mode=0):     Only heat loss to surroundings
%                    dU_i = -Q_loss_i
%
% DISCHARGING (mode=2): Q_demand drawn from TES to reheat turbine air
%                       dU_i = -Q_demand_i - Q_loss_i

T_TES_1 = U_TES_1 / (m_TES * cp_TES);
T_TES_2 = U_TES_2 / (m_TES * cp_TES);
T_TES_3 = U_TES_3 / (m_TES * cp_TES);

% Heat loss to surroundings (always active)
Q_loss_1 = UA_wall * max(0, T_TES_1 - T0);
Q_loss_2 = UA_wall * max(0, T_TES_2 - T0);
Q_loss_3 = UA_wall * max(0, T_TES_3 - T0);
Q_loss_total = Q_loss_1 + Q_loss_2 + Q_loss_3;

if mode == 1  % CHARGING
  dU_TES_1 = Q_in_1 - Q_loss_1;
  dU_TES_2 = Q_in_2 - Q_loss_2;
  dU_TES_3 = Q_in_3 - Q_loss_3;

elseif mode == 2  % DISCHARGING
  % TES supplies heat to reheaters; limit by available temperature
  Q_out_1 = min(Q_demand_1, max(0, U_TES_1/1 * 0.01)); % rate-limited
  Q_out_2 = min(Q_demand_2, max(0, U_TES_2/1 * 0.01));
  Q_out_3 = min(Q_demand_3, max(0, U_TES_3/1 * 0.01));
  dU_TES_1 = -Q_out_1 - Q_loss_1;
  dU_TES_2 = -Q_out_2 - Q_loss_2;
  dU_TES_3 = -Q_out_3 - Q_loss_3;

else  % IDLE
  dU_TES_1 = -Q_loss_1;
  dU_TES_2 = -Q_loss_2;
  dU_TES_3 = -Q_loss_3;
end

% Clamp: TES cannot go below ambient or above max temperature
U_min = m_TES * cp_TES * T0;
U_max = m_TES * cp_TES * T_TES_max;
dU_TES_1 = clamp_rate(dU_TES_1, U_TES_1, U_min, U_max);
dU_TES_2 = clamp_rate(dU_TES_2, U_TES_2, U_min, U_max);
dU_TES_3 = clamp_rate(dU_TES_3, U_TES_3, U_min, U_max);

% State of charge (based on total stored thermal energy)
U_total = U_TES_1 + U_TES_2 + U_TES_3;
U_total_min = 3 * m_TES * cp_TES * T0;
U_total_max = 3 * m_TES * cp_TES * T_TES_max;
SOC_TES = (U_total - U_total_min) / (U_total_max - U_total_min);
SOC_TES = max(0, min(1, SOC_TES));

  function r = clamp_rate(dU, U, U_lo, U_hi)
    if (U <= U_lo && dU < 0) || (U >= U_hi && dU > 0)
      r = 0;
    else
      r = dU;
    end
  end
end

== matlab function ACAES/HP_STORE/hp_store_dynamics ==
  data: m_hp input; dm_dt output; dT_dt output; T_hp input; mdot_in input; T_in input; mdot_out input; mode input; V_hp input; R_air input; cp_air input; cv_air input; gamma input; T0 input; P0 input; P_hp_min input; P_hp_max input; UA_wall_hp input; P_hp output; SOC_hp output; Ex_hp output; alarm_overpressure output; alarm_undertemp output
function [dm_dt, dT_dt, P_hp, SOC_hp, Ex_hp, alarm_overpressure, alarm_undertemp] = ...
    hp_store_dynamics(m_hp, T_hp, mdot_in, T_in, mdot_out, mode, ...
                      V_hp, R_air, cp_air, cv_air, gamma, T0, P0, ...
                      P_hp_min, P_hp_max, UA_wall_hp)
% HP_STORE_DYNAMICS: First-law open-system energy balance for HP air vessel
%
% States: m_hp [kg], T_hp [K]
% From ideal gas: P_hp = m_hp * R_air * T_hp / V_hp

% Compute current pressure from state variables
P_hp = m_hp * R_air * T_hp / V_hp;

% Safety alarms
alarm_overpressure = (P_hp > P_hp_max * 1.05);
alarm_undertemp    = (T_hp < 230);  % prevent freezing

% Wall heat transfer (idle period thermal recovery)
% During charge/discharge: adiabatic (UA_wall_hp = 0 for fast cycles)
% During idle: heat exchange with environment
if mode == 0  % IDLE
  Q_wall = UA_wall_hp * (T0 - T_hp);
else
  Q_wall = 0;
end

% Mass balance
dm_dt = mdot_in - mdot_out;

% Energy balance: dU/dt = Q_wall + mdot_in*h_in - mdot_out*h_out
% U = m*cv*T → dU/dt = cv*T*dm/dt + m*cv*dT/dt
% h_in = cp*T_in (enthalpy of incoming air)
% h_out = cp*T_hp (air leaves at bulk store temperature)
dU_dt = Q_wall + mdot_in*cp_air*T_in - mdot_out*cp_air*T_hp;

% Solve for dT_dt:
% dU/dt = cv*T_hp*(dm/dt) + m_hp*cv*(dT/dt)
if m_hp > 0.1
  dT_dt = (dU_dt - cv_air * T_hp * dm_dt) / (m_hp * cv_air);
else
  dT_dt = 0;  % prevent division by zero
end

% State of charge (pressure-based)
SOC_hp = (P_hp - P_hp_min) / (P_hp_max - P_hp_min);
SOC_hp = max(0, min(1, SOC_hp));

% Stored exergy (thermomechanical, relative to ambient)
% Simplified: Ex ≈ m * R * T0 * ln(P/P0)  (isothermal approximation)
Ex_hp = m_hp * R_air * T0 * log(max(P_hp/P0, 1.001));

% Enforce pressure bounds: stop flow if limits hit
if P_hp >= P_hp_max && mdot_in > 0
  dm_dt = min(dm_dt, 0);  % stop charging if full
  dT_dt = 0;
end
if P_hp <= P_hp_min && mdot_out > 0
  dm_dt = max(dm_dt, 0);  % stop discharging if empty
  dT_dt = 0;
end
end

== matlab function ACAES/Discharge/MATLAB Function ==
  data: P_hp input; T_exhaust output; T_hp input; T_TES_1 input; T_TES_2 input; T_TES_3 input; mdot_cmd input; enable input; gamma input; cp input; R input; T0 input; P0 input; P_throttle input; eta_turb input; eta_mech_turb input; eta_gen input; epsilon_HEX input; dP_HEX input; Kv_throttle input; tau_valve input; PR_turb_vec input; eta_turb_vec input; N_stages input; mdot_out output; W_dot_elec output; W_dot_turbine output; P_elec_actual output; Q_demand_1 output; Q_demand_2 output; Q_demand_3 output; Ex_dest_throttle output; W_dot_loss_turb output; W_dot_loss_gen output; alarm_low_TES output
function [T_exhaust, mdot_out, W_dot_elec, W_dot_turbine, ...
          P_elec_actual, Q_demand_1, Q_demand_2, Q_demand_3, ...
          Ex_dest_throttle, W_dot_loss_turb, W_dot_loss_gen, ...
          alarm_low_TES] = ...
    expansion_physics(P_hp, T_hp, T_TES_1, T_TES_2, T_TES_3, ...
                      mdot_cmd, enable, ...
                      gamma, cp, R, T0, P0, P_throttle, ...
                      eta_turb, eta_mech_turb, eta_gen, epsilon_HEX, ...
                      dP_HEX, Kv_throttle, tau_valve, ...
                      PR_turb_vec, eta_turb_vec, N_stages)
% EXPANSION_PHYSICS: 3-stage expansion with reheating from TES
% TYPE DECLARATIONS — must be first, before any logic
alarm_low_TES = false;   % declares as logical from line 1

if ~enable || P_hp < P_throttle * 1.05
  % Cannot discharge: insufficient pressure
  T_exhaust=T0; mdot_out=0; W_dot_elec=0; W_dot_turbine=0;
  P_elec_actual=0; Q_demand_1=0; Q_demand_2=0; Q_demand_3=0;
  Ex_dest_throttle=0; W_dot_loss_turb=0; W_dot_loss_gen=0;
  alarm_low_TES=false;
  return;
end

mdot = mdot_cmd;  % [kg/s]

% Safety: avoid division by zero when discharge is enabled
% but commanded mass flow is zero or negative
if mdot <= 1e-6
    T_exhaust = T0;
    mdot_out = 0;
    W_dot_elec = 0;
    W_dot_turbine = 0;
    P_elec_actual = 0;

    Q_demand_1 = 0;
    Q_demand_2 = 0;
    Q_demand_3 = 0;

    Ex_dest_throttle = 0;
    W_dot_loss_turb = 0;
    W_dot_loss_gen = 0;

    alarm_low_TES = false;
    return;
end

%% STAGE 1: THROTTLE VALVE (irreversible, isenthalpic)
% Reduces HP store pressure to turbine design-point
P_in_thr  = P_hp;
P_out_thr = P_throttle;  % regulated set-point
T_out_thr = T_hp;        % isenthalpic for ideal gas: T unchanged

% Exergy destroyed by throttle [W]
Ex_dest_throttle = mdot * R * T_hp * log(P_in_thr / P_out_thr);

%% STAGES 2-4: ALTERNATING REHEAT + EXPAND (N_stages turbine stages)
T_TES = [T_TES_3, T_TES_2, T_TES_1];  % highest TES stage used first (HPC → HPT)
T_TES_min_threshold = T0 + 10;         % TES barely warmer than ambient = depleted
alarm_low_TES = logical(any(T_TES < T_TES_min_threshold));

% Expansion pressure ratio per turbine stage (equal expansion)
PR_turb_stage = (P_throttle / P0)^(1/N_stages);
PR_turb_stage = max(1.01, PR_turb_stage);

W_dot_turb_total = 0;
Q_demand = zeros(1, N_stages);
T_stage = T_out_thr;
P_stage = P_out_thr;

for i = 1:N_stages
  % --- REHEATER (HEX): Air absorbs heat from TES ---
  C_air = mdot * cp;
  Q_available = max(0, C_air * (T_TES(i) - T_stage));  % max heat if TES at T_TES(i)
  Q_demand(i) = epsilon_HEX * Q_available;              % actual heat transferred
  T_stage = T_stage + Q_demand(i) / C_air;              % air temperature after reheater
  P_stage = P_stage * (1 - dP_HEX);                    % HEX pressure drop

  % --- TURBINE STAGE i ---
  P_out_turb = P_stage / PR_turb_stage;
  T_out_is   = T_stage * (P_out_turb / P_stage)^((gamma-1)/gamma);

  eta_is_t = interp1(PR_turb_vec, eta_turb_vec, PR_turb_stage, 'pchip', 'extrap');
  eta_is_t = max(0.40, min(0.92, eta_is_t));

  T_out_real = T_stage - eta_is_t * (T_stage - T_out_is);

  % Power from this turbine stage
  W_dot_turb_i = mdot * cp * (T_stage - T_out_real) * eta_mech_turb;
  W_dot_turb_total = W_dot_turb_total + W_dot_turb_i;

  T_stage = T_out_real;
  P_stage = P_out_turb;
end

T_exhaust     = T_stage;
mdot_out      = mdot;   % mass exits to atmosphere
W_dot_turbine = W_dot_turb_total;

% Generator conversion
W_dot_elec = W_dot_turb_total * eta_gen;
P_elec_actual = W_dot_elec;

% Losses
W_dot_ideal = mdot * cp * (T_out_thr - T0) * N_stages;  % approx ideal
W_dot_loss_turb = W_dot_turb_total - (W_dot_turb_total * eta_mech_turb);
W_dot_loss_gen  = W_dot_turb_total * eta_mech_turb * (1 - eta_gen);

% TES heat demands
Q_demand_1 = Q_demand(3);  % stage 1 TES (lowest temp, LPT reheater)
Q_demand_2 = Q_demand(2);  % stage 2 TES
Q_demand_3 = Q_demand(1);  % stage 3 TES (highest temp, HPT reheater)
end

== matlab function ACAES/DASHBOARD/MATLAB Function ==
  data: E_chg input; eta_RT output; E_dis input; E_loss_TES input; E_loss_thr input; E_loss_comp input; E_loss_turb input; E_loss_gen input; Ex_hp input; U_TES_total input; E_stored_kWh output; E_loss_total_kWh output; loss_breakdown output
function [eta_RT, E_stored_kWh, E_loss_total_kWh, loss_breakdown] = ...
    efficiency_calc(E_chg, E_dis, E_loss_TES, E_loss_thr, ...
                    E_loss_comp, E_loss_turb, E_loss_gen, Ex_hp, U_TES_total)

  % Round-trip efficiency (cumulative)
  if E_chg > 1e3
    eta_RT = E_dis / E_chg;
  else
    eta_RT = 0;
  end
  eta_RT = max(0, min(1, eta_RT));

  % Total stored energy (both stores combined)
  E_stored_kWh = (Ex_hp + U_TES_total) / 3.6e6;

  % Total losses
  E_loss_total  = E_loss_TES + E_loss_thr + E_loss_comp + E_loss_turb + E_loss_gen;
  E_loss_total_kWh = E_loss_total / 3.6e6;

  % Loss breakdown [kWh]
  loss_breakdown = [E_loss_comp, E_loss_TES, E_loss_thr, E_loss_turb, E_loss_gen] / 3.6e6;
end

== matlab function ACAES/supervisory_CTRL/MATLAB Function1 ==
  data: mode input; m_dot_chg output; P_net_W input; P_comp_rated_W input; P_turb_rated_W input; m_dot_chg_nom input; m_dot_dis_nom input; cp_air input; T0 input; gamma input; P0 input; P_hp input; m_dot_dis output; m_dot_TF output
function [m_dot_chg, m_dot_dis, m_dot_TF] = flow_commands(...
         mode, P_net_W, P_comp_rated_W, P_turb_rated_W, ...
         m_dot_chg_nom, m_dot_dis_nom, cp_air, T0, gamma, P0, P_hp)

  % During charging: flow limited by compressor rated power or surplus power
  if mode == 1
    % How much mass flow can be sustained at current HP pressure?
    PR_est = P_hp / P0;                % approximate overall pressure ratio
    w_spec = cp_air * T0 * (PR_est^((gamma-1)/gamma) - 1); % [J/kg] isentropic work/kg
    m_dot_max = P_comp_rated_W / w_spec;     % [kg/s] max flow from compressor
    m_dot_surplus = min(P_net_W, P_comp_rated_W) / w_spec; % flow from surplus
    m_dot_chg = min(m_dot_max, m_dot_surplus);
    m_dot_chg = max(0, min(m_dot_chg, m_dot_chg_nom));
  else
    m_dot_chg = 0;
  end

  % During discharging: flow limited by turbine capacity or deficit
  if mode == 2
    m_dot_dis = m_dot_dis_nom;  % constant rated flow (throttle regulates)
  else
    m_dot_dis = 0;
  end

  % TES fluid flow (balanced with air flow)
  m_dot_TF = m_dot_chg * 1005 / 1900;  % cp_air/cp_TES ratio for balanced HEX
end

== matlab function ACAES/supervisory_CTRL/MATLAB Function ==
  data: en_chg input; mode output; en_dis input; alarm input

    function mode = encode_mode(en_chg, en_dis, alarm)
      if alarm
          mode = 0;   % IDLE (emergency)
      elseif en_chg && ~en_dis
          mode = 1;   % CHARGE
      elseif en_dis && ~en_chg
          mode = 2;   % DISCHARGE
      elseif en_chg && en_dis
          % Both true (unusual): prioritize discharge to meet demand
          mode = 2;
      else
          mode = 0;   % IDLE
      end
    end

== matlab function ACAES/Subsystem/MATLAB Function ==
  data: P_net input; P_sell output; P_compress input; P_turbine input; mode input; sell_price input; buy_price input; dt input; P_buy output; cost output; revenue output

  function [P_sell, P_buy, cost, revenue] = grid_power_calc(...
           P_net, P_compress, P_turbine, mode, sell_price, buy_price, dt)
    % What power goes to/from the grid?
    % During charging:
    %   P_compress is drawn from supply (surplus used first)
    %   If surplus > P_compress: sell the rest
    %   If surplus < P_compress: buy the difference
    % During discharging:
    %   P_turbine supplements supply
    %   If supply + P_turbine > demand: sell excess
    %   If supply + P_turbine < demand: buy from grid
    
    if mode == 1   % CHARGING
      P_sell = max(0, P_net - P_compress);   % sell unused surplus
      P_buy  = max(0, P_compress - P_net);   % buy if surplus not enough
    elseif mode == 2  % DISCHARGING
      P_available = P_net + P_turbine;  % net becomes less negative
      P_sell = max(0, P_available);     % sell if still surplus
      P_buy  = max(0, -P_available);    % buy remaining deficit
    else   % IDLE
      P_sell = max(0, P_net);
      P_buy  = max(0, -P_net);
    end
    
    revenue = P_sell/1000 * sell_price * (dt/3600);   % [£] per timestep
    cost    = P_buy/1000  * buy_price  * (dt/3600);   % [£] per timestep
  end
